simulink model "mcb_microchip_pmsm_foc_sensorless_dsPIC33EP256MC506"  (R2024b)
settings: Solver=FixedStepDiscrete  StartTime=0.0  StopTime=10  FixedStep=Ts  RelTol=1e-3  EnableMultiTasking=on
InitFcn:
  | mcb_microchip_pmsm_foc_sensorless_dsPIC33_data;
undefined symbols (not defined in the file): A4, C5, D8, F1, inverter, P20, P53, P97, PI_params, Pin, pmsm, PU_System, PWM_frequency, PWMmax, Speed_openLoop_PU, Ts, Ts_speed
libraries: MCHP_Blockset x16, mcbcontrolslib x10, simulink x9, slpidlib x3, mcbpositiondecoderlib x2, mcbplantlib x1, autolibpmsmexterior x1
(part 3 of 3)

== system mcb_microchip_pmsm_foc_sensorless_dsPIC33EP256MC506/Current Control/To Matlab Host /Serial Send/SCI_Tx/Start ==
  Data : Inport
  Action Port : ActionPort  ActionPortLabel=if(u1 == 0)
  End : Constant  Value=hex2dec('53')  OutDataTypeStr=uint8
  Mux : Mux  Inputs=2
  UART Tx : MCHP_Blockset/BUS UART/UART Tx  UART_REF=2  ORDERING=None  AllOrNothing=off  SampleTime=-1  MCHP_MASTERLINK=mcb_microchip_pmsm_foc_sensorless_dsPIC33EP256MC506/Hardware Init/Microchip Master  NSend_Input=off  UART_String=off  NSend_Output=off
      settings: SourceProductName=MPLAB Device Blocks for Simulink
  wires:
  Mux/1 -> UART Tx/1
  Data/1 -> Mux/2
  End/1 -> Mux/1

== stateflow chart mcb_microchip_pmsm_foc_sensorless_dsPIC33EP256MC506/Current Control/Closed Loop Control/Open_Loop_Control/OpentoClosed/Chart ==
  state Init
    during: Mode = 0;
    SpeedCtrl = 0;
  state Align
    during: Mode = 0;
    SpeedCtrl = 0;
  state ClosedLoopFilter
    during: Mode = 2;
    SpeedCtrl = 1;
  state ClosedLoop
    during: Mode = 2;
    SpeedCtrl = 0;
  state OpenLoop
    during: Mode = 1;
    SpeedCtrl = 0;
  (default) -> Init
  ClosedLoopFilter -> Init : [En == 0]
  ClosedLoop -> Init [order 1] : [En == 0]
  Init -> Align : [En == 1]
  Align -> Init [order 1] : [En == 0]
  OpenLoop -> Init [order 2] : [En == 0]
  Align -> OpenLoop [order 2] : after(0.5,sec)
  ClosedLoop -> ClosedLoopFilter [order 2] : after(0.1,sec)
  OpenLoop -> ClosedLoop [order 1] : after(0.5,sec)[SpeedFb > Limit]
  data: Limit input fixdt(1,16,14); SpeedFb input fixdt(1,16,14); Mode output uint16; En input boolean; SpeedCtrl output uint16
